simulink model "gm_UZ_D_GaN_Inverter"  (R2021a)
settings: Solver=FixedStepDiscrete  StartTime=0.0  StopTime=300e-5  RelTol=1e-3
undefined symbols (not defined in the file or in its folder): t_clk, t_clk_sig
libraries: hdlsllib x16, simulink x12
settings Model: Creator=Michael Hoerner  LastModifiedBy=micha
settings SolverCC: AlgebraicLoopSolver=TrustRegion
settings DataIOCC: LimitDataPoints=on  SaveOutput=off  SaveTime=off
settings OptimizationCC: BlockReduction=off  ConditionallyExecuteInputs=off  DefaultParameterBehavior=Inlined  LifeSpan=inf
settings DebuggingCC: AlgebraicLoopMsg=error  InheritedTsInSrcMsg=none  SingleTaskRateTransMsg=warning  AllowSymbolicDim=off  StrictBusMsg=ErrorOnBusTreatedAsVector  SFUnexpectedBacktrackingDiag=warning  SFNoUnconditionalDefaultTransitionDiag=warning  SFExecutionAtInitializationDiag=none  SFMachineParentedDataDiag=warning  ArithmeticOperatorsInVariantConditions=warning
settings HardwareCC: ProdBitPerPointer=32  ProdBitPerSizeT=32  ProdBitPerPtrDiffT=32  ProdLargestAtomicFloat=None  ProdIntDivRoundTo=Undefined  ProdEndianess=Unspecified  ProdWordSize=32  ProdHWDeviceType=ASIC/FPGA->ASIC/FPGA  ProdEqTarget=off
settings SFSimCC: SimUseLocalCustomCode=off  CustomCodeUndefinedFunction=UseInterfaceOnly
settings RTWCC: RTWUseLocalCustomCode=off
settings CodeAppCC: StateflowObjectComments=on
settings GRTTargetCC: TargetLangStandard=C89/C90 (ANSI)
settings ConfigComp: CovScope=ReferencedModels  CovMetricSettings=dw  CovSaveCumulativeToWorkspaceVar=on  CovSaveSingleToWorkspaceVar=on  CovExternalEMLEnable=off  CovSFcnEnable=off

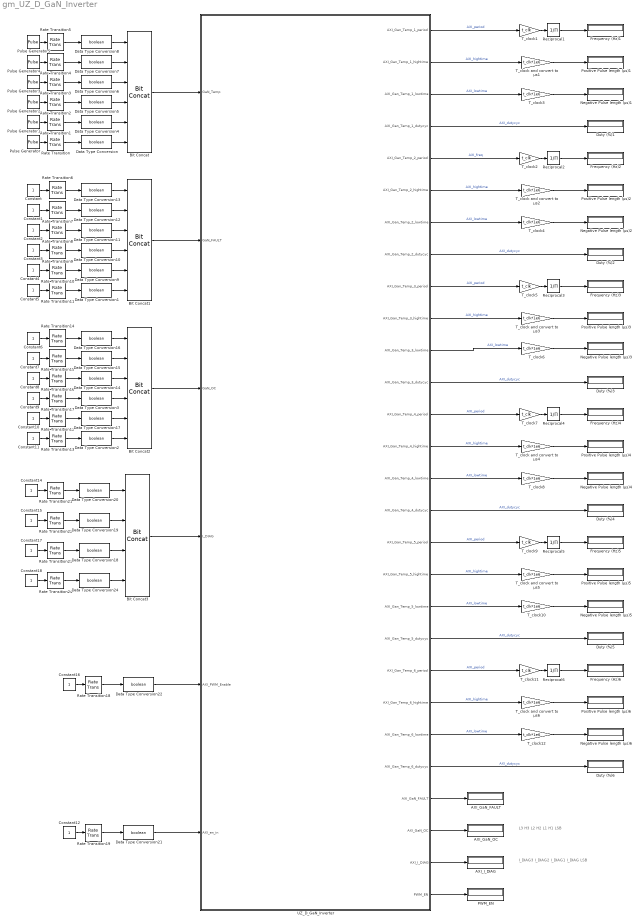
== system gm_UZ_D_GaN_Inverter ==
  note: I_DIAG3   I_DIAG2   I_DIAG1   I_DIAG
      |                                                        LSB
  note: L3   H3   L2   H2   L1   H1
      |                                   LSB
  AXI_GaN_FAULT : Display
      settings: Format=binary (Stored Integer)
  AXI_GaN_OC : Display
      settings: Format=binary (Stored Integer)
  AXI_I_DIAG : Display
      settings: Format=binary (Stored Integer)
  Bit Concat : hdlsllib/Logic and Bit Operations/Bit Concat  numInputs=6
  Bit Concat1 : hdlsllib/Logic and Bit Operations/Bit Concat  numInputs=6
  Bit Concat2 : hdlsllib/Logic and Bit Operations/Bit Concat  numInputs=6
  Bit Concat3 : hdlsllib/Logic and Bit Operations/Bit Concat  numInputs=4
  Constant{,1..12,14..18} (18 alike) : Constant
  Data Type Conversion{,1..22,24} (24 alike) : DataTypeConversion  OutDataTypeStr=boolean
  Duty (%){1..6} (6 alike) : Display
  Frequency (Hz){1..6} (6 alike) : Display
  Negative Pulse length (µs){1..6} (6 alike) : Display
  PWM_EN : Display
      settings: Format=decimal (Stored Integer)
  Positive Pulse length (µs){1..6} (6 alike) : Display
  Pulse Generator : DiscretePulseGenerator  PulseType=Time based  Period=t_clk_sig  PulseWidth=10
  Pulse Generator1 : DiscretePulseGenerator  PulseType=Time based  Period=t_clk_sig  PulseWidth=20
  Pulse Generator2 : DiscretePulseGenerator  PulseType=Time based  Period=t_clk_sig  PulseWidth=30
  Pulse Generator3 : DiscretePulseGenerator  PulseType=Time based  Period=t_clk_sig  PulseWidth=40
  Pulse Generator4 : DiscretePulseGenerator  PulseType=Time based  Period=t_clk_sig  PulseWidth=50
  Pulse Generator5 : DiscretePulseGenerator  PulseType=Time based  Period=t_clk_sig  PulseWidth=60
  Rate Transition{,1..5} (6 alike) : RateTransition  Deterministic=off  OutPortSampleTime=t_clk
  Rate Transition{6..19,21..24} (18 alike) : RateTransition  OutPortSampleTime=t_clk
  Reciprocal{1..6} (6 alike) : Product  Inputs=/
  T_clock and convert to µs{1..6} (6 alike) : Gain  Gain=t_clk*1e6
  T_clock{1..2,5,7,9,11} (6 alike) : Gain  Gain=t_clk
  T_clock{3..4,6,8,10,12} (6 alike) : Gain  Gain=t_clk*1e6
  UZ_D_GaN_Inverter : Subsystem  TreatAsAtomicUnit=on
  wires:
  Data Type Conversion21/1 -> UZ_D_GaN_Inverter/6(AXI_en_in)
  Rate Transition19/1 -> Data Type Conversion21/1
  Constant12/1 -> Rate Transition19/1
  UZ_D_GaN_Inverter/28(PWM_EN) -> PWM_EN/1
  UZ_D_GaN_Inverter/27(AXI_I_DIAG) -> AXI_I_DIAG/1
  UZ_D_GaN_Inverter/26(AXI_GaN_OC) -> AXI_GaN_OC/1
  Bit Concat3/1 -> UZ_D_GaN_Inverter/4(I_DIAG)
  Data Type Conversion24/1 -> Bit Concat3/4
  Data Type Conversion18/1 -> Bit Concat3/3
  Data Type Conversion19/1 -> Bit Concat3/2
  Data Type Conversion20/1 -> Bit Concat3/1
  Rate Transition23/1 -> Data Type Conversion18/1
  Rate Transition21/1 -> Data Type Conversion20/1
  Rate Transition24/1 -> Data Type Conversion24/1
  Constant17/1 -> Rate Transition23/1
  Constant14/1 -> Rate Transition21/1
  Rate Transition22/1 -> Data Type Conversion19/1
  Constant15/1 -> Rate Transition22/1
  Constant18/1 -> Rate Transition24/1
  Bit Concat2/1 -> UZ_D_GaN_Inverter/3(GaN_OC)
  Data Type Conversion2/1 -> Bit Concat2/6
  Constant7/1 -> Rate Transition15/1
  Rate Transition15/1 -> Data Type Conversion15/1
  Constant9/1 -> Rate Transition17/1
  Data Type Conversion17/1 -> Bit Concat2/5
  Constant10/1 -> Rate Transition12/1
  Constant11/1 -> Rate Transition13/1
  Constant8/1 -> Rate Transition16/1
  Constant6/1 -> Rate Transition14/1
  Rate Transition12/1 -> Data Type Conversion17/1
  Data Type Conversion15/1 -> Bit Concat2/2
  Data Type Conversion14/1 -> Bit Concat2/3
  Data Type Conversion3/1 -> Bit Concat2/4
  Rate Transition13/1 -> Data Type Conversion2/1
  Rate Transition14/1 -> Data Type Conversion16/1
  Rate Transition17/1 -> Data Type Conversion3/1
  Rate Transition16/1 -> Data Type Conversion14/1
  Data Type Conversion16/1 -> Bit Concat2/1
  Data Type Conversion22/1 -> UZ_D_GaN_Inverter/5(AXI_PWM_Enable)
  Rate Transition11/1 -> Data Type Conversion1/1
  Rate Transition10/1 -> Data Type Conversion9/1
  Rate Transition9/1 -> Data Type Conversion10/1
  Rate Transition8/1 -> Data Type Conversion11/1
  Rate Transition7/1 -> Data Type Conversion12/1
  Rate Transition6/1 -> Data Type Conversion13/1
  Bit Concat1/1 -> UZ_D_GaN_Inverter/2(GaN_FAULT)
  Data Type Conversion1/1 -> Bit Concat1/6
  Data Type Conversion13/1 -> Bit Concat1/1
  Data Type Conversion12/1 -> Bit Concat1/2
  Data Type Conversion9/1 -> Bit Concat1/5
  Data Type Conversion10/1 -> Bit Concat1/4
  Data Type Conversion11/1 -> Bit Concat1/3
  Data Type Conversion4/1 -> Bit Concat/5
  Data Type Conversion/1 -> Bit Concat/6
  Rate Transition5/1 -> Data Type Conversion8/1
  Rate Transition4/1 -> Data Type Conversion7/1
  Rate Transition3/1 -> Data Type Conversion6/1
  Rate Transition2/1 -> Data Type Conversion5/1
  Rate Transition1/1 -> Data Type Conversion4/1
  Bit Concat/1 -> UZ_D_GaN_Inverter/1(GaN_Temp)
  Rate Transition18/1 -> Data Type Conversion22/1
  Constant16/1 -> Rate Transition18/1
  Data Type Conversion8/1 -> Bit Concat/1
  Data Type Conversion7/1 -> Bit Concat/2
  Data Type Conversion6/1 -> Bit Concat/3
  Data Type Conversion5/1 -> Bit Concat/4
  UZ_D_GaN_Inverter/25(AXI_GaN_FAULT) -> AXI_GaN_FAULT/1
  UZ_D_GaN_Inverter/21(AXI_Gan_Temp_6_period) -> T_clock11/1  "AXI_period"
  T_clock and convert to µs6/1 -> Positive Pulse length (µs)6/1
  UZ_D_GaN_Inverter/22(AXI_Gan_Temp_6_hightime) -> T_clock and convert to µs6/1  "AXI_hightime"
  T_clock12/1 -> Negative Pulse length (µs)6/1
  Reciprocal6/1 -> Frequency (Hz)6/1
  UZ_D_GaN_Inverter/24(AXI_Gan_Temp_6_dutycyc) -> Duty (%)6/1  "AXI_dutycyc"
  T_clock11/1 -> Reciprocal6/1
  UZ_D_GaN_Inverter/23(AXI_Gan_Temp_6_lowtime) -> T_clock12/1  "AXI_lowtime"
  UZ_D_GaN_Inverter/17(AXI_Gan_Temp_5_period) -> T_clock9/1  "AXI_period"
  T_clock and convert to µs5/1 -> Positive Pulse length (µs)5/1
  UZ_D_GaN_Inverter/18(AXI_Gan_Temp_5_hightime) -> T_clock and convert to µs5/1  "AXI_hightime"
  T_clock10/1 -> Negative Pulse length (µs)5/1
  Reciprocal5/1 -> Frequency (Hz)5/1
  UZ_D_GaN_Inverter/20(AXI_Gan_Temp_5_dutycyc) -> Duty (%)5/1  "AXI_dutycyc"
  T_clock9/1 -> Reciprocal5/1
  UZ_D_GaN_Inverter/19(AXI_Gan_Temp_5_lowtime) -> T_clock10/1  "AXI_lowtime"
  UZ_D_GaN_Inverter/13(AXI_Gan_Temp_4_period) -> T_clock7/1  "AXI_period"
  T_clock and convert to µs4/1 -> Positive Pulse length (µs)4/1
  UZ_D_GaN_Inverter/14(AXI_Gan_Temp_4_hightime) -> T_clock and convert to µs4/1  "AXI_hightime"
  T_clock8/1 -> Negative Pulse length (µs)4/1
  Reciprocal4/1 -> Frequency (Hz)4/1
  UZ_D_GaN_Inverter/16(AXI_Gan_Temp_4_dutycyc) -> Duty (%)4/1  "AXI_dutycyc"
  T_clock7/1 -> Reciprocal4/1
  UZ_D_GaN_Inverter/15(AXI_Gan_Temp_4_lowtime) -> T_clock8/1  "AXI_lowtime"
  UZ_D_GaN_Inverter/9(AXI_Gan_Temp_3_period) -> T_clock5/1  "AXI_period"
  T_clock and convert to µs3/1 -> Positive Pulse length (µs)3/1
  UZ_D_GaN_Inverter/10(AXI_Gan_Temp_3_hightime) -> T_clock and convert to µs3/1  "AXI_hightime"
  T_clock6/1 -> Negative Pulse length (µs)3/1
  Reciprocal3/1 -> Frequency (Hz)3/1
  UZ_D_GaN_Inverter/12(AXI_Gan_Temp_3_dutycyc) -> Duty (%)3/1  "AXI_dutycyc"
  T_clock5/1 -> Reciprocal3/1
  UZ_D_GaN_Inverter/11(AXI_Gan_Temp_3_lowtime) -> T_clock6/1  "AXI_lowtime"
  UZ_D_GaN_Inverter/5(AXI_Gan_Temp_2_period) -> T_clock2/1  "AXI_freq"
  T_clock and convert to µs2/1 -> Positive Pulse length (µs)2/1
  UZ_D_GaN_Inverter/6(AXI_Gan_Temp_2_hightime) -> T_clock and convert to µs2/1  "AXI_hightime"
  T_clock4/1 -> Negative Pulse length (µs)2/1
  Reciprocal2/1 -> Frequency (Hz)2/1
  UZ_D_GaN_Inverter/8(AXI_Gan_Temp_2_dutycyc) -> Duty (%)2/1  "AXI_dutycyc"
  T_clock2/1 -> Reciprocal2/1
  UZ_D_GaN_Inverter/7(AXI_Gan_Temp_2_lowtime) -> T_clock4/1  "AXI_lowtime"
  UZ_D_GaN_Inverter/4(AXI_Gan_Temp_1_dutycyc) -> Duty (%)1/1  "AXI_dutycyc"
  UZ_D_GaN_Inverter/1(AXI_Gan_Temp_1_period) -> T_clock1/1  "AXI_period"
  T_clock1/1 -> Reciprocal1/1
  UZ_D_GaN_Inverter/2(AXI_Gan_Temp_1_hightime) -> T_clock and convert to µs1/1  "AXI_hightime"
  UZ_D_GaN_Inverter/3(AXI_Gan_Temp_1_lowtime) -> T_clock3/1  "AXI_lowtime"
  Reciprocal1/1 -> Frequency (Hz)1/1
  T_clock3/1 -> Negative Pulse length (µs)1/1
  T_clock and convert to µs1/1 -> Positive Pulse length (µs)1/1
  Constant5/1 -> Rate Transition11/1
  Constant4/1 -> Rate Transition10/1
  Constant3/1 -> Rate Transition9/1
  Constant2/1 -> Rate Transition8/1
  Constant1/1 -> Rate Transition7/1
  Constant/1 -> Rate Transition6/1
  Rate Transition/1 -> Data Type Conversion/1
  Pulse Generator5/1 -> Rate Transition5/1
  Pulse Generator4/1 -> Rate Transition4/1
  Pulse Generator3/1 -> Rate Transition3/1
  Pulse Generator2/1 -> Rate Transition2/1
  Pulse Generator1/1 -> Rate Transition1/1
  Pulse Generator/1 -> Rate Transition/1

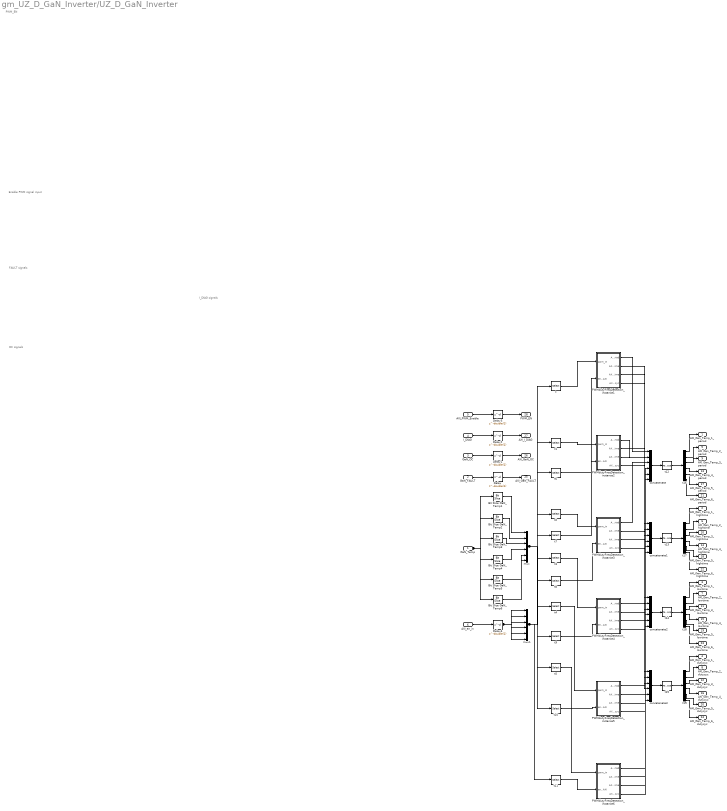
== system gm_UZ_D_GaN_Inverter/UZ_D_GaN_Inverter ==
  note: PWM_EN
  note: I_DIAG signals
  note: FAULT signals
  note: OC signals
  note: Enable PWM signal input
  GaN_Temp : Inport  OutDataTypeStr=fixdt(0, 6, 0)  PortDimensions=1  SampleTime=1e-08
  GaN_FAULT : Inport  Port=2  OutDataTypeStr=fixdt(0, 6, 0)  PortDimensions=1  SampleTime=1e-08
  GaN_OC : Inport  Port=3  OutDataTypeStr=fixdt(0, 6, 0)  PortDimensions=1  SampleTime=1e-08
  I_DIAG : Inport  Port=4  OutDataTypeStr=fixdt(0, 4, 0)  PortDimensions=1  SampleTime=1e-08
  AXI_PWM_Enable : Inport  Port=5  OutDataTypeStr=boolean  PortDimensions=1  SampleTime=1e-08
  AXI_en_in : Inport  Port=6  OutDataTypeStr=boolean  PortDimensions=1  SampleTime=1e-08
  Bit Slice GaN_Temp1 : hdlsllib/Logic and Bit Operations/Bit Slice  lidx=double(0)  ridx=double(0)
      settings: SourceProductBaseCode=SL
  Bit Slice GaN_Temp2 : hdlsllib/Logic and Bit Operations/Bit Slice  lidx=double(1)  ridx=double(1)
      settings: SourceProductBaseCode=SL
  Bit Slice GaN_Temp3 : hdlsllib/Logic and Bit Operations/Bit Slice  lidx=double(2)  ridx=double(2)
      settings: SourceProductBaseCode=SL
  Bit Slice GaN_Temp4 : hdlsllib/Logic and Bit Operations/Bit Slice  lidx=double(3)  ridx=double(3)
      settings: SourceProductBaseCode=SL
  Bit Slice GaN_Temp5 : hdlsllib/Logic and Bit Operations/Bit Slice  lidx=double(4)  ridx=double(4)
      settings: SourceProductBaseCode=SL
  Bit Slice GaN_Temp6 : hdlsllib/Logic and Bit Operations/Bit Slice  lidx=double(5)  ridx=double(5)
      settings: SourceProductBaseCode=SL
  Delay{,1..4} (5 alike) : Delay  DelayLength=double(1)  InitialCondition=0  SampleTime=1e-08
  PWMdutyFreqDetection_instance1 : Subsystem
  PWMdutyFreqDetection_instance2 : Subsystem
  PWMdutyFreqDetection_instance3 : Subsystem
  PWMdutyFreqDetection_instance4 : Subsystem
  PWMdutyFreqDetection_instance5 : Subsystem
  PWMdutyFreqDetection_instance6 : Subsystem
  concatenate{,1..3} (4 alike) : Concatenate  NumInputs=6
  mux : Mux  Inputs=6
  mux1 : Mux  Inputs=6
  t : Selector  SampleTime=1e-08  IndexOptions=Index vector (dialog)  Indices=double(1)  OutputSizes=1
  t1 : Selector  SampleTime=1e-08  IndexOptions=Index vector (dialog)  Indices=double(2)  OutputSizes=1
  t10 : Selector  SampleTime=1e-08  IndexOptions=Index vector (dialog)  Indices=double(5)  OutputSizes=1
  t11 : Selector  SampleTime=1e-08  IndexOptions=Index vector (dialog)  Indices=double(6)  OutputSizes=1
  t{12..15} (4 alike) : Reshape
  t{16..19} (4 alike) : Demux  Outputs=6
  t2 : Selector  SampleTime=1e-08  IndexOptions=Index vector (dialog)  Indices=double(3)  OutputSizes=1
  t3 : Selector  SampleTime=1e-08  IndexOptions=Index vector (dialog)  Indices=double(4)  OutputSizes=1
  t4 : Selector  SampleTime=1e-08  IndexOptions=Index vector (dialog)  Indices=double(5)  OutputSizes=1
  t5 : Selector  SampleTime=1e-08  IndexOptions=Index vector (dialog)  Indices=double(6)  OutputSizes=1
  t6 : Selector  SampleTime=1e-08  IndexOptions=Index vector (dialog)  Indices=double(1)  OutputSizes=1
  t7 : Selector  SampleTime=1e-08  IndexOptions=Index vector (dialog)  Indices=double(2)  OutputSizes=1
  t8 : Selector  SampleTime=1e-08  IndexOptions=Index vector (dialog)  Indices=double(3)  OutputSizes=1
  t9 : Selector  SampleTime=1e-08  IndexOptions=Index vector (dialog)  Indices=double(4)  OutputSizes=1
  AXI_Gan_Temp_1_period : Outport  PortDimensions=1  SampleTime=1e-08  VectorParamsAs1DForOutWhenUnconnected=off
  AXI_Gan_Temp_1_hightime : Outport  Port=2  PortDimensions=1  SampleTime=1e-08  VectorParamsAs1DForOutWhenUnconnected=off
  AXI_Gan_Temp_1_lowtime : Outport  Port=3  PortDimensions=1  SampleTime=1e-08  VectorParamsAs1DForOutWhenUnconnected=off
  AXI_Gan_Temp_1_dutycyc : Outport  Port=4  PortDimensions=1  SampleTime=1e-08  VectorParamsAs1DForOutWhenUnconnected=off
  AXI_Gan_Temp_2_period : Outport  Port=5  PortDimensions=1  SampleTime=1e-08  VectorParamsAs1DForOutWhenUnconnected=off
  AXI_Gan_Temp_2_hightime : Outport  Port=6  PortDimensions=1  SampleTime=1e-08  VectorParamsAs1DForOutWhenUnconnected=off
  AXI_Gan_Temp_2_lowtime : Outport  Port=7  PortDimensions=1  SampleTime=1e-08  VectorParamsAs1DForOutWhenUnconnected=off
  AXI_Gan_Temp_2_dutycyc : Outport  Port=8  PortDimensions=1  SampleTime=1e-08  VectorParamsAs1DForOutWhenUnconnected=off
  AXI_Gan_Temp_3_period : Outport  Port=9  PortDimensions=1  SampleTime=1e-08  VectorParamsAs1DForOutWhenUnconnected=off
  AXI_Gan_Temp_3_hightime : Outport  Port=10  PortDimensions=1  SampleTime=1e-08  VectorParamsAs1DForOutWhenUnconnected=off
  AXI_Gan_Temp_3_lowtime : Outport  Port=11  PortDimensions=1  SampleTime=1e-08  VectorParamsAs1DForOutWhenUnconnected=off
  AXI_Gan_Temp_3_dutycyc : Outport  Port=12  PortDimensions=1  SampleTime=1e-08  VectorParamsAs1DForOutWhenUnconnected=off
  AXI_Gan_Temp_4_period : Outport  Port=13  PortDimensions=1  SampleTime=1e-08  VectorParamsAs1DForOutWhenUnconnected=off
  AXI_Gan_Temp_4_hightime : Outport  Port=14  PortDimensions=1  SampleTime=1e-08  VectorParamsAs1DForOutWhenUnconnected=off
  AXI_Gan_Temp_4_lowtime : Outport  Port=15  PortDimensions=1  SampleTime=1e-08  VectorParamsAs1DForOutWhenUnconnected=off
  AXI_Gan_Temp_4_dutycyc : Outport  Port=16  PortDimensions=1  SampleTime=1e-08  VectorParamsAs1DForOutWhenUnconnected=off
  AXI_Gan_Temp_5_period : Outport  Port=17  PortDimensions=1  SampleTime=1e-08  VectorParamsAs1DForOutWhenUnconnected=off
  AXI_Gan_Temp_5_hightime : Outport  Port=18  PortDimensions=1  SampleTime=1e-08  VectorParamsAs1DForOutWhenUnconnected=off
  AXI_Gan_Temp_5_lowtime : Outport  Port=19  PortDimensions=1  SampleTime=1e-08  VectorParamsAs1DForOutWhenUnconnected=off
  AXI_Gan_Temp_5_dutycyc : Outport  Port=20  PortDimensions=1  SampleTime=1e-08  VectorParamsAs1DForOutWhenUnconnected=off
  AXI_Gan_Temp_6_period : Outport  Port=21  PortDimensions=1  SampleTime=1e-08  VectorParamsAs1DForOutWhenUnconnected=off
  AXI_Gan_Temp_6_hightime : Outport  Port=22  PortDimensions=1  SampleTime=1e-08  VectorParamsAs1DForOutWhenUnconnected=off
  AXI_Gan_Temp_6_lowtime : Outport  Port=23  PortDimensions=1  SampleTime=1e-08  VectorParamsAs1DForOutWhenUnconnected=off
  AXI_Gan_Temp_6_dutycyc : Outport  Port=24  PortDimensions=1  SampleTime=1e-08  VectorParamsAs1DForOutWhenUnconnected=off
  AXI_GaN_FAULT : Outport  Port=25  PortDimensions=1  SampleTime=1e-08  VectorParamsAs1DForOutWhenUnconnected=off
  AXI_GaN_OC : Outport  Port=26  PortDimensions=1  SampleTime=1e-08  VectorParamsAs1DForOutWhenUnconnected=off
  AXI_I_DIAG : Outport  Port=27  PortDimensions=1  SampleTime=1e-08  VectorParamsAs1DForOutWhenUnconnected=off
  PWM_EN : Outport  Port=28  PortDimensions=1  SampleTime=1e-08  VectorParamsAs1DForOutWhenUnconnected=off
  wires:
  GaN_Temp/1 -> Bit Slice GaN_Temp6/1, Bit Slice GaN_Temp5/1, Bit Slice GaN_Temp4/1, Bit Slice GaN_Temp3/1, Bit Slice GaN_Temp2/1, Bit Slice GaN_Temp1/1
  GaN_FAULT/1 -> Delay/1
  GaN_OC/1 -> Delay1/1
  I_DIAG/1 -> Delay2/1
  AXI_PWM_Enable/1 -> Delay3/1
  AXI_en_in/1 -> Delay4/1
  Bit Slice GaN_Temp1/1 -> mux/1
  Bit Slice GaN_Temp2/1 -> mux/2
  Bit Slice GaN_Temp3/1 -> mux/3
  Bit Slice GaN_Temp4/1 -> mux/4
  Bit Slice GaN_Temp5/1 -> mux/5
  Bit Slice GaN_Temp6/1 -> mux/6
  Delay/1 -> AXI_GaN_FAULT/1
  Delay1/1 -> AXI_GaN_OC/1
  Delay2/1 -> AXI_I_DIAG/1
  Delay3/1 -> PWM_EN/1
  Delay4/1 -> mux1/6, mux1/5, mux1/4, mux1/3, mux1/2, mux1/1
  mux/1 -> t5/1, t4/1, t3/1, t2/1, t1/1, t/1
  mux1/1 -> t11/1, t10/1, t9/1, t8/1, t7/1, t6/1
  t12/1 -> t16/1
  t13/1 -> t17/1
  t14/1 -> t18/1
  t15/1 -> t19/1
  t/1 -> PWMdutyFreqDetection_instance1/1(pwm_in)
  t1/1 -> PWMdutyFreqDetection_instance2/1(pwm_in)
  t2/1 -> PWMdutyFreqDetection_instance3/1(pwm_in)
  t3/1 -> PWMdutyFreqDetection_instance4/1(pwm_in)
  t4/1 -> PWMdutyFreqDetection_instance5/1(pwm_in)
  t5/1 -> PWMdutyFreqDetection_instance6/1(pwm_in)
  t6/1 -> PWMdutyFreqDetection_instance1/2(en_in_AXI)
  t7/1 -> PWMdutyFreqDetection_instance2/2(en_in_AXI)
  t8/1 -> PWMdutyFreqDetection_instance3/2(en_in_AXI)
  t9/1 -> PWMdutyFreqDetection_instance4/2(en_in_AXI)
  t10/1 -> PWMdutyFreqDetection_instance5/2(en_in_AXI)
  t11/1 -> PWMdutyFreqDetection_instance6/2(en_in_AXI)
  concatenate/1 -> t12/1
  PWMdutyFreqDetection_instance1/1(AXI_period) -> concatenate/1
  PWMdutyFreqDetection_instance2/1(AXI_period) -> concatenate/2
  PWMdutyFreqDetection_instance3/1(AXI_period) -> concatenate/3
  PWMdutyFreqDetection_instance4/1(AXI_period) -> concatenate/4
  PWMdutyFreqDetection_instance5/1(AXI_period) -> concatenate/5
  PWMdutyFreqDetection_instance6/1(AXI_period) -> concatenate/6
  concatenate1/1 -> t13/1
  PWMdutyFreqDetection_instance1/2(AXI_hightime) -> concatenate1/1
  PWMdutyFreqDetection_instance2/2(AXI_hightime) -> concatenate1/2
  PWMdutyFreqDetection_instance3/2(AXI_hightime) -> concatenate1/3
  PWMdutyFreqDetection_instance4/2(AXI_hightime) -> concatenate1/4
  PWMdutyFreqDetection_instance5/2(AXI_hightime) -> concatenate1/5
  PWMdutyFreqDetection_instance6/2(AXI_hightime) -> concatenate1/6
  concatenate2/1 -> t14/1
  PWMdutyFreqDetection_instance1/3(AXI_lowtime) -> concatenate2/1
  PWMdutyFreqDetection_instance2/3(AXI_lowtime) -> concatenate2/2
  PWMdutyFreqDetection_instance3/3(AXI_lowtime) -> concatenate2/3
  PWMdutyFreqDetection_instance4/3(AXI_lowtime) -> concatenate2/4
  PWMdutyFreqDetection_instance5/3(AXI_lowtime) -> concatenate2/5
  PWMdutyFreqDetection_instance6/3(AXI_lowtime) -> concatenate2/6
  concatenate3/1 -> t15/1
  PWMdutyFreqDetection_instance1/4(AXI_dutycyc) -> concatenate3/1
  PWMdutyFreqDetection_instance2/4(AXI_dutycyc) -> concatenate3/2
  PWMdutyFreqDetection_instance3/4(AXI_dutycyc) -> concatenate3/3
  PWMdutyFreqDetection_instance4/4(AXI_dutycyc) -> concatenate3/4
  PWMdutyFreqDetection_instance5/4(AXI_dutycyc) -> concatenate3/5
  PWMdutyFreqDetection_instance6/4(AXI_dutycyc) -> concatenate3/6
  t16/1 -> AXI_Gan_Temp_1_period/1
  t16/2 -> AXI_Gan_Temp_2_period/1
  t16/3 -> AXI_Gan_Temp_3_period/1
  t16/4 -> AXI_Gan_Temp_4_period/1
  t16/5 -> AXI_Gan_Temp_5_period/1
  t16/6 -> AXI_Gan_Temp_6_period/1
  t17/1 -> AXI_Gan_Temp_1_hightime/1
  t17/2 -> AXI_Gan_Temp_2_hightime/1
  t17/3 -> AXI_Gan_Temp_3_hightime/1
  t17/4 -> AXI_Gan_Temp_4_hightime/1
  t17/5 -> AXI_Gan_Temp_5_hightime/1
  t17/6 -> AXI_Gan_Temp_6_hightime/1
  t18/1 -> AXI_Gan_Temp_1_lowtime/1
  t18/2 -> AXI_Gan_Temp_2_lowtime/1
  t18/3 -> AXI_Gan_Temp_3_lowtime/1
  t18/4 -> AXI_Gan_Temp_4_lowtime/1
  t18/5 -> AXI_Gan_Temp_5_lowtime/1
  t18/6 -> AXI_Gan_Temp_6_lowtime/1
  t19/1 -> AXI_Gan_Temp_1_dutycyc/1
  t19/2 -> AXI_Gan_Temp_2_dutycyc/1
  t19/3 -> AXI_Gan_Temp_3_dutycyc/1
  t19/4 -> AXI_Gan_Temp_4_dutycyc/1
  t19/5 -> AXI_Gan_Temp_5_dutycyc/1
  t19/6 -> AXI_Gan_Temp_6_dutycyc/1

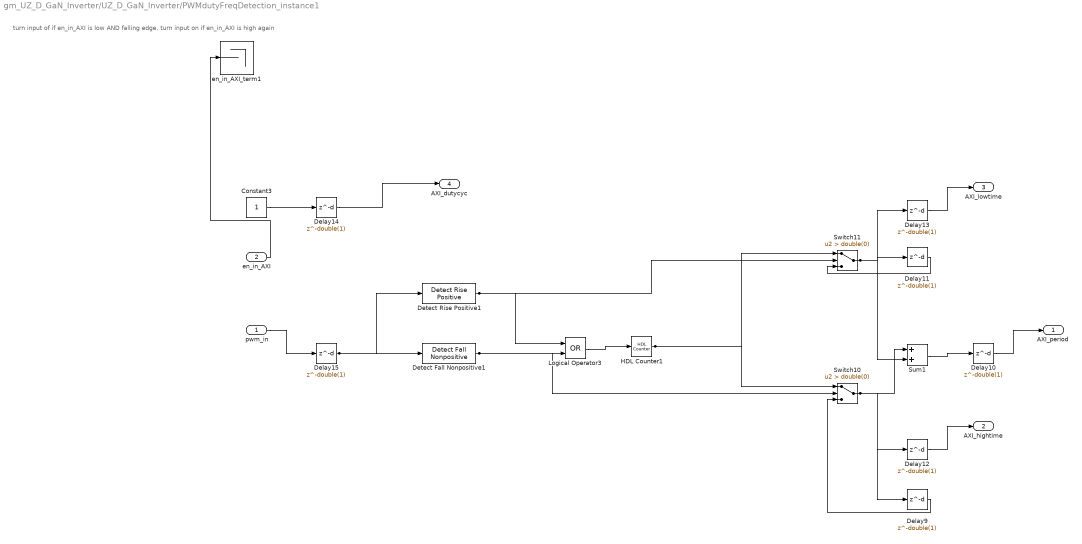
== system gm_UZ_D_GaN_Inverter/UZ_D_GaN_Inverter/PWMdutyFreqDetection_instance1 ==
  note: turn input of if en_in_AXI is low AND falling edge, turn input on if en_in_AXI is high again
  pwm_in : Inport  OutDataTypeStr=fixdt(0, 1, 0)  PortDimensions=1  SampleTime=1e-08
  en_in_AXI : Inport  Port=2  OutDataTypeStr=boolean  PortDimensions=1  SampleTime=1e-08
  Constant3 : Constant  OutDataTypeStr=uint32  SampleTime=1e-08
  Delay{9..15} (7 alike) : Delay  DelayLength=double(1)  InitialCondition=0  SampleTime=1e-08
  Detect Fall Nonpositive1 : simulink/Logic and Bit Operations/Detect Fall Nonpositive  vinit=0  OutDataTypeStr=boolean
      settings: SourceProductBaseCode=SL
  Detect Rise Positive1 : simulink/Logic and Bit Operations/Detect Rise Positive  vinit=0  OutDataTypeStr=boolean
  HDL Counter1 : hdlsllib/Sources/HDL Counter  CountType=Count limited  CountInit=double(1)  CountStep=double(1)  CountMax=double(2500000)  CountFromType=Initial value  CountFrom=double(1)  CountResetPort=on  CountLoadPort=off  CountEnbPort=off  CountDirPort=off  CountHitOutputPort=off  CountDataType=Unsigned  CountWordLen=32  CountFracLen=0  CountSampTime=1e-08
  Logical Operator3 : Logic  Operator=OR  AllPortsSameDT=off  OutDataTypeStr=boolean  SampleTime=1e-08
  Sum1 : Sum  AccumDataTypeStr=uint32  OutDataTypeStr=uint32  SampleTime=1e-08
  Switch10 : Switch  Criteria=u2 > Threshold  Threshold=double(0)  OutDataTypeStr=uint32  SampleTime=1e-08
  Switch11 : Switch  Criteria=u2 > Threshold  Threshold=double(0)  OutDataTypeStr=uint32  SampleTime=1e-08
  en_in_AXI_term1 : Terminator
  AXI_period : Outport  SampleTime=1e-08
  AXI_hightime : Outport  Port=2  SampleTime=1e-08
  AXI_lowtime : Outport  Port=3  SampleTime=1e-08
  AXI_dutycyc : Outport  Port=4  SampleTime=1e-08
  wires:
  pwm_in/1 -> Delay15/1
  en_in_AXI/1 -> en_in_AXI_term1/1
  Switch11/1 -> Sum1/2, Delay11/1, Delay13/1
  Switch10/1 -> Sum1/1, Delay12/1, Delay9/1
  Sum1/1 -> Delay10/1
  Logical Operator3/1 -> HDL Counter1/1
  HDL Counter1/1 -> Switch10/1, Switch11/1
  Detect Rise Positive1/1 -> Logical Operator3/1, Switch11/2
  Detect Fall Nonpositive1/1 -> Logical Operator3/2, Switch10/2
  Delay9/1 -> Switch10/3
  Delay15/1 -> Detect Fall Nonpositive1/1, Detect Rise Positive1/1
  Delay14/1 -> AXI_dutycyc/1
  Delay13/1 -> AXI_lowtime/1
  Delay12/1 -> AXI_hightime/1
  Delay11/1 -> Switch11/3
  Delay10/1 -> AXI_period/1
  Constant3/1 -> Delay14/1

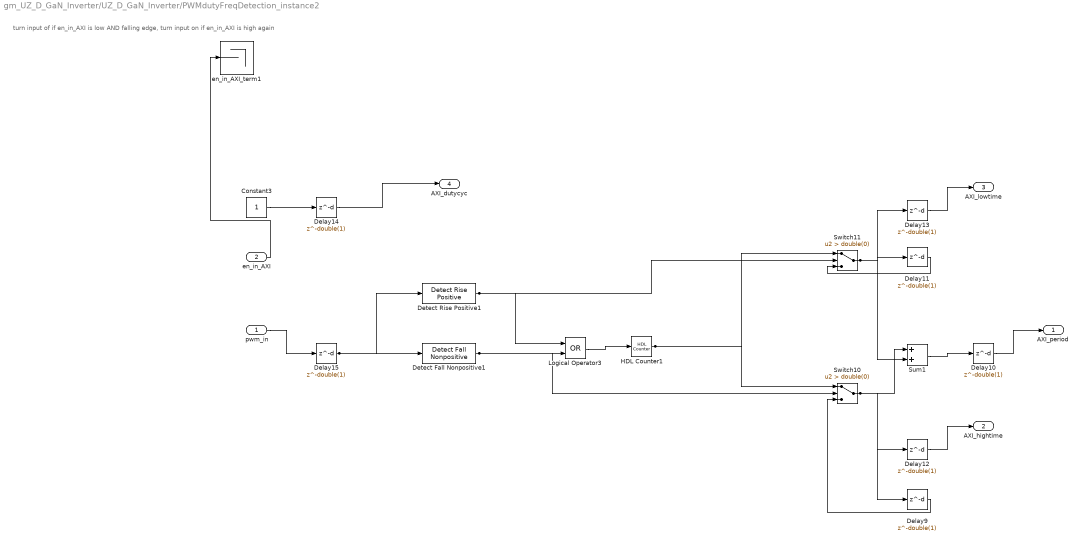
== system gm_UZ_D_GaN_Inverter/UZ_D_GaN_Inverter/PWMdutyFreqDetection_instance2 ==
  note: turn input of if en_in_AXI is low AND falling edge, turn input on if en_in_AXI is high again
  pwm_in : Inport  OutDataTypeStr=fixdt(0, 1, 0)  PortDimensions=1  SampleTime=1e-08
  en_in_AXI : Inport  Port=2  OutDataTypeStr=boolean  PortDimensions=1  SampleTime=1e-08
  Constant3 : Constant  OutDataTypeStr=uint32  SampleTime=1e-08
  Delay{9..15} (7 alike) : Delay  DelayLength=double(1)  InitialCondition=0  SampleTime=1e-08
  Detect Fall Nonpositive1 : simulink/Logic and Bit Operations/Detect Fall Nonpositive  vinit=0  OutDataTypeStr=boolean
      settings: SourceProductBaseCode=SL
  Detect Rise Positive1 : simulink/Logic and Bit Operations/Detect Rise Positive  vinit=0  OutDataTypeStr=boolean
  HDL Counter1 : hdlsllib/Sources/HDL Counter  CountType=Count limited  CountInit=double(1)  CountStep=double(1)  CountMax=double(2500000)  CountFromType=Initial value  CountFrom=double(1)  CountResetPort=on  CountLoadPort=off  CountEnbPort=off  CountDirPort=off  CountHitOutputPort=off  CountDataType=Unsigned  CountWordLen=32  CountFracLen=0  CountSampTime=1e-08
  Logical Operator3 : Logic  Operator=OR  AllPortsSameDT=off  OutDataTypeStr=boolean  SampleTime=1e-08
  Sum1 : Sum  AccumDataTypeStr=uint32  OutDataTypeStr=uint32  SampleTime=1e-08
  Switch10 : Switch  Criteria=u2 > Threshold  Threshold=double(0)  OutDataTypeStr=uint32  SampleTime=1e-08
  Switch11 : Switch  Criteria=u2 > Threshold  Threshold=double(0)  OutDataTypeStr=uint32  SampleTime=1e-08
  en_in_AXI_term1 : Terminator
  AXI_period : Outport  SampleTime=1e-08
  AXI_hightime : Outport  Port=2  SampleTime=1e-08
  AXI_lowtime : Outport  Port=3  SampleTime=1e-08
  AXI_dutycyc : Outport  Port=4  SampleTime=1e-08
  wires:
  Constant3/1 -> Delay14/1
  Delay10/1 -> AXI_period/1
  Delay11/1 -> Switch11/3
  Delay12/1 -> AXI_hightime/1
  Delay13/1 -> AXI_lowtime/1
  Delay14/1 -> AXI_dutycyc/1
  Delay15/1 -> Detect Rise Positive1/1, Detect Fall Nonpositive1/1
  Delay9/1 -> Switch10/3
  Detect Fall Nonpositive1/1 -> Switch10/2, Logical Operator3/2
  Detect Rise Positive1/1 -> Switch11/2, Logical Operator3/1
  HDL Counter1/1 -> Switch11/1, Switch10/1
  Logical Operator3/1 -> HDL Counter1/1
  Sum1/1 -> Delay10/1
  Switch10/1 -> Delay9/1, Delay12/1, Sum1/1
  Switch11/1 -> Delay13/1, Delay11/1, Sum1/2
  en_in_AXI/1 -> en_in_AXI_term1/1
  pwm_in/1 -> Delay15/1

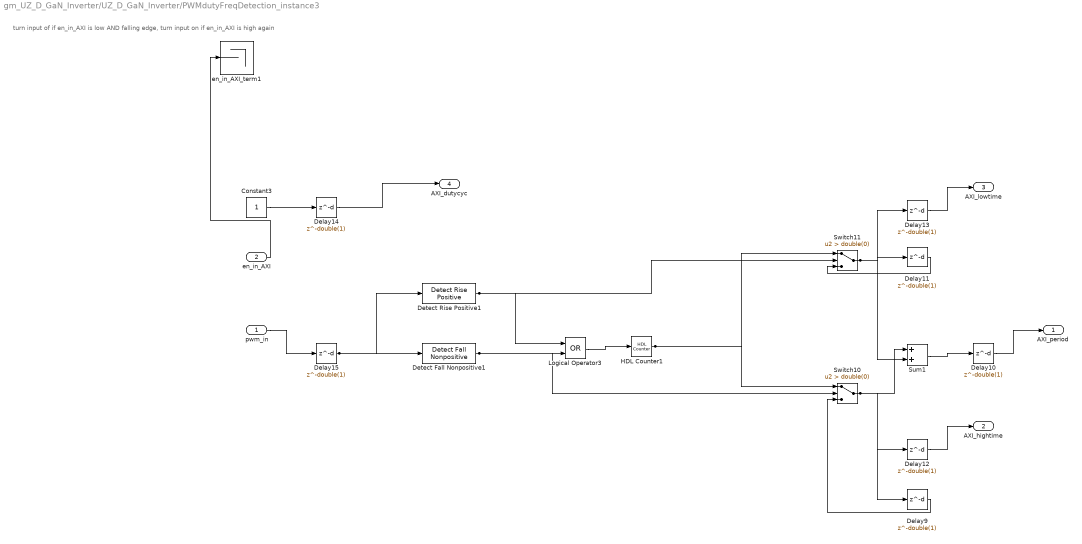
== system gm_UZ_D_GaN_Inverter/UZ_D_GaN_Inverter/PWMdutyFreqDetection_instance3 ==
  note: turn input of if en_in_AXI is low AND falling edge, turn input on if en_in_AXI is high again
  pwm_in : Inport  OutDataTypeStr=fixdt(0, 1, 0)  PortDimensions=1  SampleTime=1e-08
  en_in_AXI : Inport  Port=2  OutDataTypeStr=boolean  PortDimensions=1  SampleTime=1e-08
  Constant3 : Constant  OutDataTypeStr=uint32  SampleTime=1e-08
  Delay{9..15} (7 alike) : Delay  DelayLength=double(1)  InitialCondition=0  SampleTime=1e-08
  Detect Fall Nonpositive1 : simulink/Logic and Bit Operations/Detect Fall Nonpositive  vinit=0  OutDataTypeStr=boolean
      settings: SourceProductBaseCode=SL
  Detect Rise Positive1 : simulink/Logic and Bit Operations/Detect Rise Positive  vinit=0  OutDataTypeStr=boolean
  HDL Counter1 : hdlsllib/Sources/HDL Counter  CountType=Count limited  CountInit=double(1)  CountStep=double(1)  CountMax=double(2500000)  CountFromType=Initial value  CountFrom=double(1)  CountResetPort=on  CountLoadPort=off  CountEnbPort=off  CountDirPort=off  CountHitOutputPort=off  CountDataType=Unsigned  CountWordLen=32  CountFracLen=0  CountSampTime=1e-08
  Logical Operator3 : Logic  Operator=OR  AllPortsSameDT=off  OutDataTypeStr=boolean  SampleTime=1e-08
  Sum1 : Sum  AccumDataTypeStr=uint32  OutDataTypeStr=uint32  SampleTime=1e-08
  Switch10 : Switch  Criteria=u2 > Threshold  Threshold=double(0)  OutDataTypeStr=uint32  SampleTime=1e-08
  Switch11 : Switch  Criteria=u2 > Threshold  Threshold=double(0)  OutDataTypeStr=uint32  SampleTime=1e-08
  en_in_AXI_term1 : Terminator
  AXI_period : Outport  SampleTime=1e-08
  AXI_hightime : Outport  Port=2  SampleTime=1e-08
  AXI_lowtime : Outport  Port=3  SampleTime=1e-08
  AXI_dutycyc : Outport  Port=4  SampleTime=1e-08
  wires:
  Constant3/1 -> Delay14/1
  Delay10/1 -> AXI_period/1
  Delay11/1 -> Switch11/3
  Delay12/1 -> AXI_hightime/1
  Delay13/1 -> AXI_lowtime/1
  Delay14/1 -> AXI_dutycyc/1
  Delay15/1 -> Detect Rise Positive1/1, Detect Fall Nonpositive1/1
  Delay9/1 -> Switch10/3
  Detect Fall Nonpositive1/1 -> Switch10/2, Logical Operator3/2
  Detect Rise Positive1/1 -> Switch11/2, Logical Operator3/1
  HDL Counter1/1 -> Switch11/1, Switch10/1
  Logical Operator3/1 -> HDL Counter1/1
  Sum1/1 -> Delay10/1
  Switch10/1 -> Delay9/1, Delay12/1, Sum1/1
  Switch11/1 -> Delay13/1, Delay11/1, Sum1/2
  en_in_AXI/1 -> en_in_AXI_term1/1
  pwm_in/1 -> Delay15/1

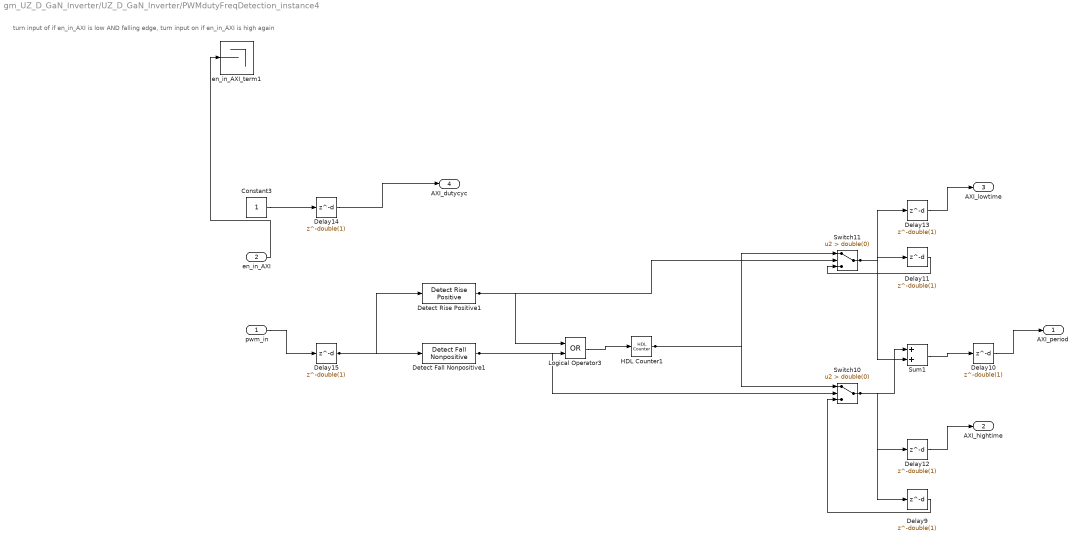
== system gm_UZ_D_GaN_Inverter/UZ_D_GaN_Inverter/PWMdutyFreqDetection_instance4 ==
  note: turn input of if en_in_AXI is low AND falling edge, turn input on if en_in_AXI is high again
  pwm_in : Inport  OutDataTypeStr=fixdt(0, 1, 0)  PortDimensions=1  SampleTime=1e-08
  en_in_AXI : Inport  Port=2  OutDataTypeStr=boolean  PortDimensions=1  SampleTime=1e-08
  Constant3 : Constant  OutDataTypeStr=uint32  SampleTime=1e-08
  Delay{9..15} (7 alike) : Delay  DelayLength=double(1)  InitialCondition=0  SampleTime=1e-08
  Detect Fall Nonpositive1 : simulink/Logic and Bit Operations/Detect Fall Nonpositive  vinit=0  OutDataTypeStr=boolean
      settings: SourceProductBaseCode=SL
  Detect Rise Positive1 : simulink/Logic and Bit Operations/Detect Rise Positive  vinit=0  OutDataTypeStr=boolean
  HDL Counter1 : hdlsllib/Sources/HDL Counter  CountType=Count limited  CountInit=double(1)  CountStep=double(1)  CountMax=double(2500000)  CountFromType=Initial value  CountFrom=double(1)  CountResetPort=on  CountLoadPort=off  CountEnbPort=off  CountDirPort=off  CountHitOutputPort=off  CountDataType=Unsigned  CountWordLen=32  CountFracLen=0  CountSampTime=1e-08
  Logical Operator3 : Logic  Operator=OR  AllPortsSameDT=off  OutDataTypeStr=boolean  SampleTime=1e-08
  Sum1 : Sum  AccumDataTypeStr=uint32  OutDataTypeStr=uint32  SampleTime=1e-08
  Switch10 : Switch  Criteria=u2 > Threshold  Threshold=double(0)  OutDataTypeStr=uint32  SampleTime=1e-08
  Switch11 : Switch  Criteria=u2 > Threshold  Threshold=double(0)  OutDataTypeStr=uint32  SampleTime=1e-08
  en_in_AXI_term1 : Terminator
  AXI_period : Outport  SampleTime=1e-08
  AXI_hightime : Outport  Port=2  SampleTime=1e-08
  AXI_lowtime : Outport  Port=3  SampleTime=1e-08
  AXI_dutycyc : Outport  Port=4  SampleTime=1e-08
  wires:
  Constant3/1 -> Delay14/1
  Delay10/1 -> AXI_period/1
  Delay11/1 -> Switch11/3
  Delay12/1 -> AXI_hightime/1
  Delay13/1 -> AXI_lowtime/1
  Delay14/1 -> AXI_dutycyc/1
  Delay15/1 -> Detect Rise Positive1/1, Detect Fall Nonpositive1/1
  Delay9/1 -> Switch10/3
  Detect Fall Nonpositive1/1 -> Switch10/2, Logical Operator3/2
  Detect Rise Positive1/1 -> Switch11/2, Logical Operator3/1
  HDL Counter1/1 -> Switch11/1, Switch10/1
  Logical Operator3/1 -> HDL Counter1/1
  Sum1/1 -> Delay10/1
  Switch10/1 -> Delay9/1, Delay12/1, Sum1/1
  Switch11/1 -> Delay13/1, Delay11/1, Sum1/2
  en_in_AXI/1 -> en_in_AXI_term1/1
  pwm_in/1 -> Delay15/1

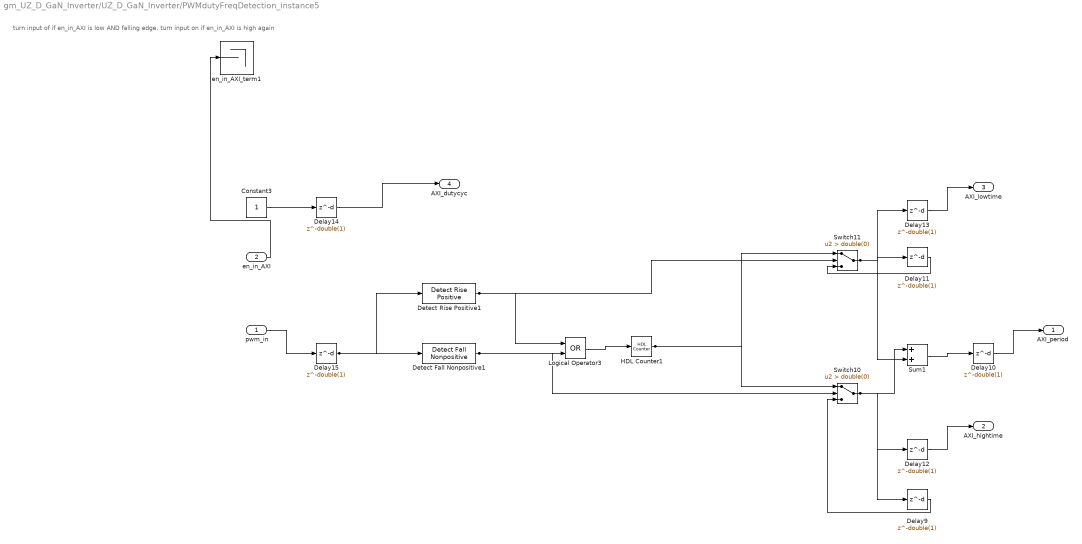
== system gm_UZ_D_GaN_Inverter/UZ_D_GaN_Inverter/PWMdutyFreqDetection_instance5 ==
  note: turn input of if en_in_AXI is low AND falling edge, turn input on if en_in_AXI is high again
  pwm_in : Inport  OutDataTypeStr=fixdt(0, 1, 0)  PortDimensions=1  SampleTime=1e-08
  en_in_AXI : Inport  Port=2  OutDataTypeStr=boolean  PortDimensions=1  SampleTime=1e-08
  Constant3 : Constant  OutDataTypeStr=uint32  SampleTime=1e-08
  Delay{9..15} (7 alike) : Delay  DelayLength=double(1)  InitialCondition=0  SampleTime=1e-08
  Detect Fall Nonpositive1 : simulink/Logic and Bit Operations/Detect Fall Nonpositive  vinit=0  OutDataTypeStr=boolean
      settings: SourceProductBaseCode=SL
  Detect Rise Positive1 : simulink/Logic and Bit Operations/Detect Rise Positive  vinit=0  OutDataTypeStr=boolean
  HDL Counter1 : hdlsllib/Sources/HDL Counter  CountType=Count limited  CountInit=double(1)  CountStep=double(1)  CountMax=double(2500000)  CountFromType=Initial value  CountFrom=double(1)  CountResetPort=on  CountLoadPort=off  CountEnbPort=off  CountDirPort=off  CountHitOutputPort=off  CountDataType=Unsigned  CountWordLen=32  CountFracLen=0  CountSampTime=1e-08
  Logical Operator3 : Logic  Operator=OR  AllPortsSameDT=off  OutDataTypeStr=boolean  SampleTime=1e-08
  Sum1 : Sum  AccumDataTypeStr=uint32  OutDataTypeStr=uint32  SampleTime=1e-08
  Switch10 : Switch  Criteria=u2 > Threshold  Threshold=double(0)  OutDataTypeStr=uint32  SampleTime=1e-08
  Switch11 : Switch  Criteria=u2 > Threshold  Threshold=double(0)  OutDataTypeStr=uint32  SampleTime=1e-08
  en_in_AXI_term1 : Terminator
  AXI_period : Outport  SampleTime=1e-08
  AXI_hightime : Outport  Port=2  SampleTime=1e-08
  AXI_lowtime : Outport  Port=3  SampleTime=1e-08
  AXI_dutycyc : Outport  Port=4  SampleTime=1e-08
  wires:
  Constant3/1 -> Delay14/1
  Delay10/1 -> AXI_period/1
  Delay11/1 -> Switch11/3
  Delay12/1 -> AXI_hightime/1
  Delay13/1 -> AXI_lowtime/1
  Delay14/1 -> AXI_dutycyc/1
  Delay15/1 -> Detect Rise Positive1/1, Detect Fall Nonpositive1/1
  Delay9/1 -> Switch10/3
  Detect Fall Nonpositive1/1 -> Switch10/2, Logical Operator3/2
  Detect Rise Positive1/1 -> Switch11/2, Logical Operator3/1
  HDL Counter1/1 -> Switch11/1, Switch10/1
  Logical Operator3/1 -> HDL Counter1/1
  Sum1/1 -> Delay10/1
  Switch10/1 -> Delay9/1, Delay12/1, Sum1/1
  Switch11/1 -> Delay13/1, Delay11/1, Sum1/2
  en_in_AXI/1 -> en_in_AXI_term1/1
  pwm_in/1 -> Delay15/1

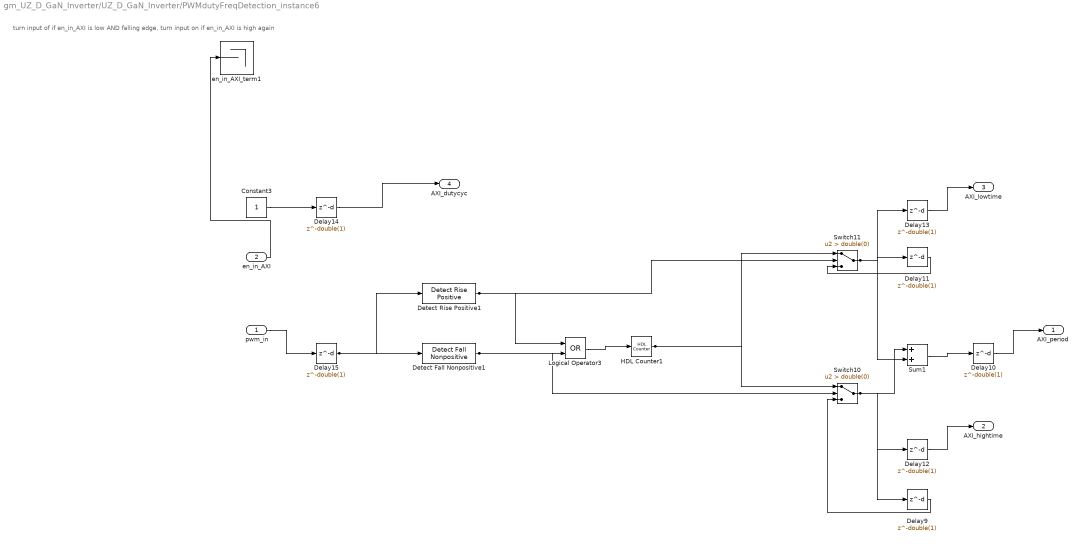
== system gm_UZ_D_GaN_Inverter/UZ_D_GaN_Inverter/PWMdutyFreqDetection_instance6 ==
  note: turn input of if en_in_AXI is low AND falling edge, turn input on if en_in_AXI is high again
  pwm_in : Inport  OutDataTypeStr=fixdt(0, 1, 0)  PortDimensions=1  SampleTime=1e-08
  en_in_AXI : Inport  Port=2  OutDataTypeStr=boolean  PortDimensions=1  SampleTime=1e-08
  Constant3 : Constant  OutDataTypeStr=uint32  SampleTime=1e-08
  Delay{9..15} (7 alike) : Delay  DelayLength=double(1)  InitialCondition=0  SampleTime=1e-08
  Detect Fall Nonpositive1 : simulink/Logic and Bit Operations/Detect Fall Nonpositive  vinit=0  OutDataTypeStr=boolean
      settings: SourceProductBaseCode=SL
  Detect Rise Positive1 : simulink/Logic and Bit Operations/Detect Rise Positive  vinit=0  OutDataTypeStr=boolean
  HDL Counter1 : hdlsllib/Sources/HDL Counter  CountType=Count limited  CountInit=double(1)  CountStep=double(1)  CountMax=double(2500000)  CountFromType=Initial value  CountFrom=double(1)  CountResetPort=on  CountLoadPort=off  CountEnbPort=off  CountDirPort=off  CountHitOutputPort=off  CountDataType=Unsigned  CountWordLen=32  CountFracLen=0  CountSampTime=1e-08
  Logical Operator3 : Logic  Operator=OR  AllPortsSameDT=off  OutDataTypeStr=boolean  SampleTime=1e-08
  Sum1 : Sum  AccumDataTypeStr=uint32  OutDataTypeStr=uint32  SampleTime=1e-08
  Switch10 : Switch  Criteria=u2 > Threshold  Threshold=double(0)  OutDataTypeStr=uint32  SampleTime=1e-08
  Switch11 : Switch  Criteria=u2 > Threshold  Threshold=double(0)  OutDataTypeStr=uint32  SampleTime=1e-08
  en_in_AXI_term1 : Terminator
  AXI_period : Outport  SampleTime=1e-08
  AXI_hightime : Outport  Port=2  SampleTime=1e-08
  AXI_lowtime : Outport  Port=3  SampleTime=1e-08
  AXI_dutycyc : Outport  Port=4  SampleTime=1e-08
  wires:
  Constant3/1 -> Delay14/1
  Delay10/1 -> AXI_period/1
  Delay11/1 -> Switch11/3
  Delay12/1 -> AXI_hightime/1
  Delay13/1 -> AXI_lowtime/1
  Delay14/1 -> AXI_dutycyc/1
  Delay15/1 -> Detect Rise Positive1/1, Detect Fall Nonpositive1/1
  Delay9/1 -> Switch10/3
  Detect Fall Nonpositive1/1 -> Switch10/2, Logical Operator3/2
  Detect Rise Positive1/1 -> Switch11/2, Logical Operator3/1
  HDL Counter1/1 -> Switch11/1, Switch10/1
  Logical Operator3/1 -> HDL Counter1/1
  Sum1/1 -> Delay10/1
  Switch10/1 -> Delay9/1, Delay12/1, Sum1/1
  Switch11/1 -> Delay13/1, Delay11/1, Sum1/2
  en_in_AXI/1 -> en_in_AXI_term1/1
  pwm_in/1 -> Delay15/1
